simulink model "nms_model_nonlin"  (R2020a)
settings: Solver=VariableStepAuto  StartTime=0.0  StopTime=7  FixedStep=0.0001  MaxStep=.01  RelTol=1e-4  AbsTol=1e-6
values from neighbouring files (symbols this model uses):
  animFrameRate = 10    [runmodel.m]
  dt_visual = -1    [NMScontrol.m]    (also in runmodel.m = 0.001)
  g = params.g    [NMPCcostFunction.m]    (also in dynamicsNMPC.m = 9.81)
  m = parametersOpt(1)    [CGBgreybox.m]    (also in NMPCcostFunction.m = params.m)
  params = setupParamsStruct(parametersOpt, dt, controlParams)    [CGBcontrol.m]    (also in CGBgreybox.m = setupParamsStruct(parametersOpt); computationTime.m = setupParamsStruct(ParametersOpt, Qy, yref, dt))
undefined symbols (not defined in the file or in its folder): footMass, hatLeftHipToCenterDistWidth, hatMass, initialTargetAngle, legMass, LongDelay, LongLoopDelay, LPreStimBFSHinit, LPreStimGASinit, LPreStimGLUinit, LPreStimHABinit, LPreStimHADinit, LPreStimHAMinit, LPreStimHFLinit, LPreStimRFinit, LPreStimSOLinit, LPreStimTAinit, LPreStimVASinit, LTargetAngleInit, LTargetAngleRInit, MidDelay, RPreStimBFSHinit, RPreStimGASinit, RPreStimGLUinit, RPreStimHABinit, RPreStimHADinit, RPreStimHAMinit, RPreStimHFLinit, RPreStimRFinit, RPreStimSOLinit, RPreStimTAinit, RPreStimVASinit, RTargetAngleInit, RTargetAngleRInit, shankLength, shankMass, ShortDelay, termination_height, thetaHATref, thighLength, thighMass, totalMass, X, Y, Z
libraries: NeuroMuscularLibrary x113, nesl_utility x30, sm_lib x24, simulink x3
(part 3 of 5)

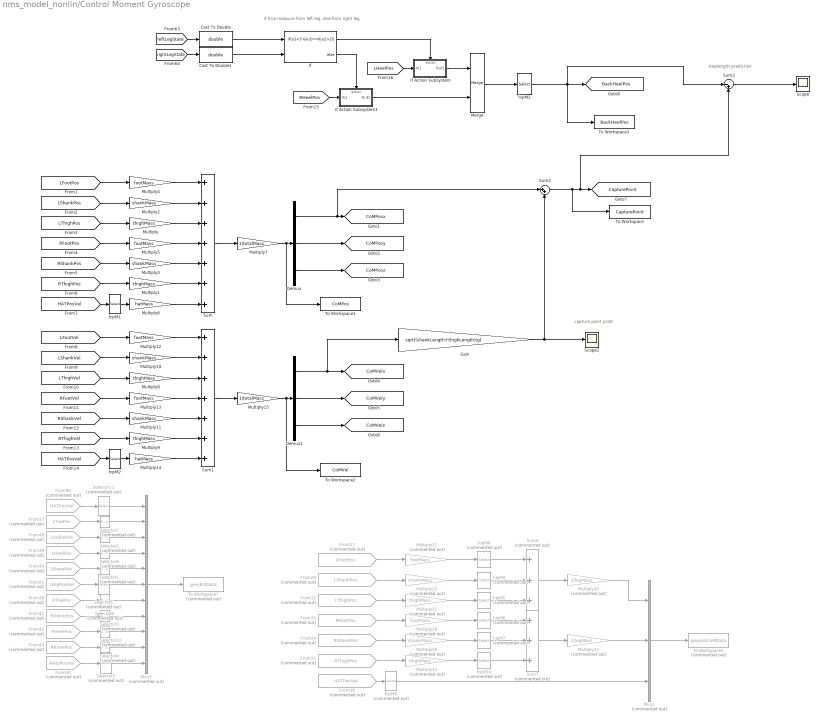
== system nms_model_nonlin/Control Moment Gyroscope ==
  note: capture point pratt
  note: steplength prediction
  note: if true measure from left leg, else from right leg
  Cast To Double : DataTypeConversion  OutDataTypeStr=double
  Cast To Double1 : DataTypeConversion  OutDataTypeStr=double
  Demux : Demux  Outputs=3
  Demux1 : Demux  Outputs=3
  From27 : From  Commented=on  GotoTag=LFootPos  TagVisibility=global
  From28 : From  Commented=on  GotoTag=LShankPos  TagVisibility=global
  From32 : From  Commented=on  GotoTag=LThighPos  TagVisibility=global
  From33 : From  Commented=on  GotoTag=RFootPos  TagVisibility=global
  From34 : From  Commented=on  GotoTag=RShankPos  TagVisibility=global
  From35 : From  Commented=on  GotoTag=RThighPos  TagVisibility=global
  From36 : From  Commented=on  GotoTag=HATPosVel  TagVisibility=global
  From37 : From  Commented=on  GotoTag=LToePos  TagVisibility=global
      settings: CloseFcn=tagdialog Close
  From38 : From  Commented=on  GotoTag=RToePos  TagVisibility=global
      settings: CloseFcn=tagdialog Close
  From39 : From  Commented=on  GotoTag=LHeelPos  TagVisibility=global
      settings: CloseFcn=tagdialog Close
  From40 : From  Commented=on  GotoTag=RHipPosVel  TagVisibility=global
  From41 : From  Commented=on  GotoTag=RAnklePos  TagVisibility=global
      settings: CloseFcn=tagdialog Close
  From42 : From  Commented=on  GotoTag=RHeelPos  TagVisibility=global
      settings: CloseFcn=tagdialog Close
  From43 : From  Commented=on  GotoTag=RKneePos  TagVisibility=global
      settings: CloseFcn=tagdialog Close
  From48 : From  Commented=on  GotoTag=LAnklePos  TagVisibility=global
      settings: CloseFcn=tagdialog Close
  From49 : From  Commented=on  GotoTag=LKneePos  TagVisibility=global
      settings: CloseFcn=tagdialog Close
  From90 : From  Commented=on  GotoTag=HATPosVel  TagVisibility=global
  From91 : From  Commented=on  GotoTag=LHipPosVel  TagVisibility=global
  Gain : Gain  Gain=sqrt((shankLength+thighLength)/g)
  If : If  NumInputs=2  IfExpression=u1<3 &(u2==0|u2>2)
  If Action Subsystem : Subsystem  TreatAsAtomicUnit=on
  If Action Subsystem1 : Subsystem  TreatAsAtomicUnit=on
  Merge : Merge
  Multiply{,1,8..9} (4 alike) : Gain  Gain=thighMass
  Multiply{2..3,10..11} (4 alike) : Gain  Gain=shankMass
  Multiply{4..5,12..13} (4 alike) : Gain  Gain=footMass
  Multiply14 : Gain  Gain=hatMass
  Multiply15 : Gain  Gain=1/totalMass
  Multiply25 : Gain  Commented=on  Gain=shankMass
  Multiply26 : Gain  Commented=on  Gain=shankMass
  Multiply27 : Gain  Commented=on  Gain=footMass
  Multiply28 : Gain  Commented=on  Gain=footMass
  Multiply30 : Gain  Commented=on  Gain=1/legMass
  Multiply31 : Gain  Commented=on  Gain=thighMass
  Multiply32 : Gain  Commented=on  Gain=thighMass
  Multiply33 : Gain  Commented=on  Gain=1/legMass
  Multiply6 : Gain  Gain=hatMass
  Multiply7 : Gain  Gain=1/totalMass
  Mux2 : Mux  Commented=on  Inputs=3
  Mux3 : Mux  Commented=on  Inputs=11
  Scope : Scope
  Scope1 : Scope
  Selector{1..4,7..10} (8 alike) : Selector  Commented=on  InputPortWidth=3  IndexOptions=Index vector (dialog)  Indices=[1 3]  OutputSizes=1
  Selector11 : Selector  Commented=on  InputPortWidth=6  IndexOptions=Index vector (dialog)  Indices=[1,3]  OutputSizes=1
  Selector5 : Selector  Commented=on  InputPortWidth=6  IndexOptions=Index vector (dialog)  Indices=[1,3]  OutputSizes=1
  Selector6 : Selector  Commented=on  InputPortWidth=6  IndexOptions=Index vector (dialog)  Indices=[1,3]  OutputSizes=1
  Sum : Sum  Inputs=+++++++
  Sum1 : Sum  Inputs=+++++++
  Sum2 : Sum  Inputs=|++
  Sum3 : Sum  Inputs=|-+
  Sum6 : Sum  Commented=on  Inputs=+++
  Sum7 : Sum  Commented=on  Inputs=+++
  To Workspace : ToWorkspace  VariableName=CapturePoint  SaveFormat=Structure With Time  SampleTime=0.01
  To Workspace1 : ToWorkspace  VariableName=CoMPos  SaveFormat=Structure With Time  SampleTime=0.01
  To Workspace2 : ToWorkspace  VariableName=CoMVel  SaveFormat=Structure With Time  SampleTime=0.01
  To Workspace3 : ToWorkspace  VariableName=BackHeelPos  SaveFormat=Structure With Time  SampleTime=0.01
  To Workspace5 : ToWorkspace  Commented=on  VariableName=greyEstCoMData  SaveFormat=Structure With Time  SampleTime=dt_visual
  To Workspace7 : ToWorkspace  Commented=on  VariableName=greyEstData  SaveFormat=Structure With Time  SampleTime=dt_visual
  hipM1 : Selector  InputPortWidth=6  IndexOptions=Index vector (dialog)  Indices=[1:3]  OutputSizes=1
  hipM{4..7,9..10} (6 alike) : Selector  Commented=on  InputPortWidth=3  IndexOptions=Index vector (dialog)  Indices=[1;3]  OutputSizes=1
  hipM2 : Selector  InputPortWidth=6  IndexOptions=Index vector (dialog)  Indices=[4:6]  OutputSizes=1
  hipM3 : Selector  InputPortWidth=3  IndexOptions=Index vector (dialog)  Indices=1  OutputSizes=1
  hipM8 : Selector  Commented=on  InputPortWidth=6  IndexOptions=Index vector (dialog)  Indices=[1;3]  OutputSizes=1
  tag scope: BackHeelPos=global, CapturePoint=global, CoMPosx=global, CoMPosy=global, CoMPosz=global, CoMVelx=global, CoMVely=global, CoMVelz=global
  wires:
  [LFootPos] -> Multiply4/1
  [LShankPos] -> Multiply2/1
  [RFootPos] -> Multiply5/1
  [LThighPos] -> Multiply/1
  [RShankPos] -> Multiply3/1
  [RThighPos] -> Multiply1/1
  [HATPosVel] -> hipM1/1
  Multiply4/1 -> Sum/1
  Multiply2/1 -> Sum/2
  Multiply/1 -> Sum/3
  Multiply5/1 -> Sum/4
  Multiply3/1 -> Sum/5
  Multiply1/1 -> Sum/6
  Multiply6/1 -> Sum/7
  Sum/1 -> Multiply7/1
  hipM1/1 -> Multiply6/1
  Multiply7/1 -> To Workspace1/1, Demux/1
  Demux/2 -> [CoMPosy]
  Demux/3 -> [CoMPosz]
  Demux/1 -> Sum2/1, [CoMPosx]
  Demux1/2 -> [CoMVely]
  hipM2/1 -> Multiply14/1
  Multiply14/1 -> Sum1/7
  Multiply12/1 -> Sum1/1
  Multiply8/1 -> Sum1/3
  [LThighVel] -> Multiply8/1
  [LShankVel] -> Multiply10/1
  Multiply13/1 -> Sum1/4
  [HATPosVel] -> hipM2/1
  Multiply11/1 -> Sum1/5
  Multiply15/1 -> To Workspace2/1, Demux1/1
  Multiply9/1 -> Sum1/6
  Demux1/3 -> [CoMVelz]
  [RFootVel] -> Multiply13/1
  Multiply10/1 -> Sum1/2
  [RThighVel] -> Multiply9/1
  Sum1/1 -> Multiply15/1
  [LFootVel] -> Multiply12/1
  [RShankVel] -> Multiply11/1
  Demux1/1 -> Gain/1, [CoMVelx]
  Gain/1 -> Sum2/2, Scope1/1
  Sum2/1 -> To Workspace/1, Sum3/2, [CapturePoint]
  [rightLegState] -> Cast To Double1/1
  [leftLegState] -> Cast To Double/1
  Cast To Double/1 -> If/1
  Cast To Double1/1 -> If/2
  If/1 -> If Action Subsystem/Action
  If/2 -> If Action Subsystem1/Action
  If Action Subsystem/1(Out1) -> Merge/1
  If Action Subsystem1/1(Out1) -> Merge/2
  [RHeelPos] -> If Action Subsystem1/1(In1)
  [LHeelPos] -> If Action Subsystem/1(In1)
  Merge/1 -> hipM3/1
  Sum3/1 -> Scope/1
  hipM3/1 -> Sum3/1, [BackHeelPos], To Workspace3/1
  hipM7/1 -> Sum7/2
  hipM8/1 -> Mux2/3
  hipM6/1 -> Sum7/1
  From33/1 -> Multiply28/1
  From35/1 -> Multiply32/1
  hipM9/1 -> Sum6/1
  From36/1 -> hipM8/1
  From32/1 -> Multiply31/1
  Multiply25/1 -> hipM4/1
  Multiply33/1 -> Mux2/2
  Sum6/1 -> Multiply30/1
  From28/1 -> Multiply25/1
  hipM4/1 -> Sum6/2
  Multiply27/1 -> hipM9/1
  From27/1 -> Multiply27/1
  Multiply31/1 -> hipM5/1
  Mux2/1 -> To Workspace5/1
  Sum7/1 -> Multiply33/1
  Multiply30/1 -> Mux2/1
  hipM5/1 -> Sum6/3
  hipM10/1 -> Sum7/3
  Multiply28/1 -> hipM6/1
  Multiply26/1 -> hipM7/1
  From34/1 -> Multiply26/1
  Multiply32/1 -> hipM10/1
  From40/1 -> Selector5/1
  From39/1 -> Selector9/1
  Selector9/1 -> Mux3/4
  Selector10/1 -> Mux3/9
  From42/1 -> Selector10/1
  From43/1 -> Selector4/1
  Selector5/1 -> Mux3/11
  Selector8/1 -> Mux3/7
  From48/1 -> Selector2/1
  Selector2/1 -> Mux3/3
  Selector6/1 -> Mux3/6
  Selector7/1 -> Mux3/2
  Selector11/1 -> Mux3/1
  Selector4/1 -> Mux3/10
  Selector3/1 -> Mux3/8
  From41/1 -> Selector3/1
  From37/1 -> Selector7/1
  From91/1 -> Selector6/1
  Mux3/1 -> To Workspace7/1
  From38/1 -> Selector8/1
  From90/1 -> Selector11/1
  From49/1 -> Selector1/1
  Selector1/1 -> Mux3/5

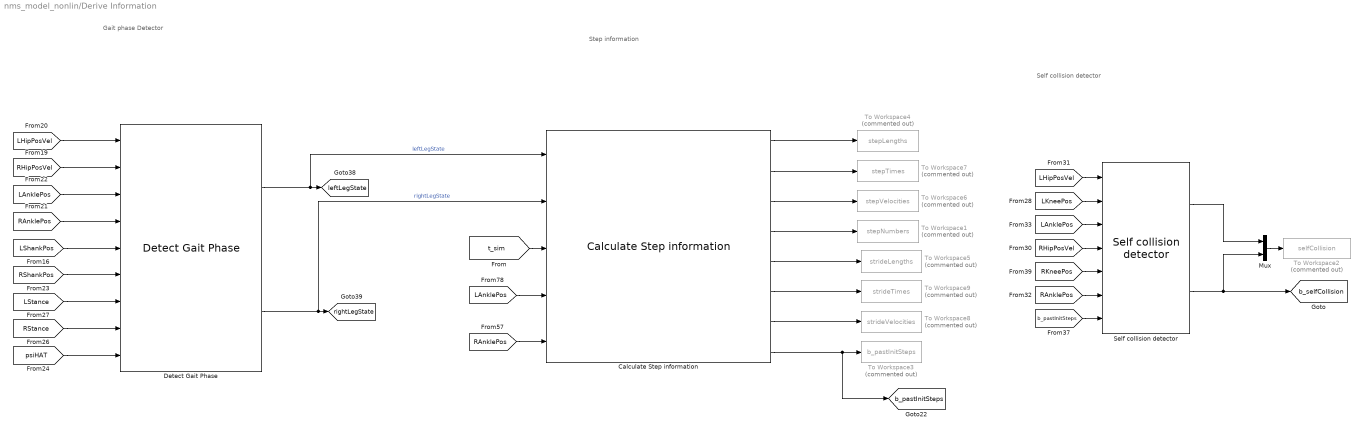
== system nms_model_nonlin/Derive Information ==
  note: Self collision detector
  note: Gait phase Detector
  note: Step information
  Calculate Step information : NeuroMuscularLibrary/Calculate Step information  initiationSteps=innerOptSettings.initiationSteps
  Detect Gait Phase : NeuroMuscularLibrary/Detect Gait Phase  SystemSampleTime=-1  Latency=0  AutoFrameSizeCalculation=off
  Mux : Mux  Inputs=2
  Self collision detector : NeuroMuscularLibrary/Self collision detector  maxDist=innerOptSettings.minLimbDistance
  To Workspace1 : ToWorkspace  Commented=on  VariableName=stepNumbers  SaveFormat=Structure With Time  SampleTime=-1
  To Workspace2 : ToWorkspace  Commented=on  VariableName=selfCollision  SaveFormat=Structure With Time  SampleTime=dt_visual
  To Workspace3 : ToWorkspace  Commented=on  VariableName=b_pastInitSteps  SaveFormat=Structure With Time  SampleTime=dt_visual
  To Workspace4 : ToWorkspace  Commented=on  VariableName=stepLengths  SaveFormat=Structure With Time  SampleTime=-1
  To Workspace5 : ToWorkspace  Commented=on  VariableName=strideLengths  SaveFormat=Structure With Time  SampleTime=-1
  To Workspace6 : ToWorkspace  Commented=on  VariableName=stepVelocities  SaveFormat=Structure With Time  SampleTime=-1
  To Workspace7 : ToWorkspace  Commented=on  VariableName=stepTimes  SaveFormat=Structure With Time  SampleTime=-1
  To Workspace8 : ToWorkspace  Commented=on  VariableName=strideVelocities  SaveFormat=Structure With Time  SampleTime=-1
  To Workspace9 : ToWorkspace  Commented=on  VariableName=strideTimes  SaveFormat=Structure With Time  SampleTime=-1
  tag scope: b_pastInitSteps=global, b_selfCollision=global, leftLegState=global, rightLegState=global
  wires:
  [RHipPosVel] -> Detect Gait Phase/2
  [LKneePos] -> Self collision detector/2
  [RHipPosVel] -> Self collision detector/4
  Mux/1 -> To Workspace2/1
  Self collision detector/2 -> [b_selfCollision], Mux/2
  [RAnklePos] -> Self collision detector/6
  Detect Gait Phase/1 -> Calculate Step information/1, [leftLegState]  "leftLegState"
  [LHipPosVel] -> Detect Gait Phase/1
  Self collision detector/1 -> Mux/1
  Detect Gait Phase/2 -> Calculate Step information/2, [rightLegState]  "rightLegState"
  [LHipPosVel] -> Self collision detector/1
  [b_pastInitSteps] -> Self collision detector/7
  [RStance] -> Detect Gait Phase/8
  [LStance] -> Detect Gait Phase/7
  [RShankPos] -> Detect Gait Phase/6
  [RAnklePos] -> Detect Gait Phase/4
  [psiHAT] -> Detect Gait Phase/9
  [RKneePos] -> Self collision detector/5
  [LAnklePos] -> Self collision detector/3
  [LShankPos] -> Detect Gait Phase/5
  [LAnklePos] -> Detect Gait Phase/3
  [RAnklePos] -> Calculate Step information/5
  Calculate Step information/1 -> To Workspace4/1
  Calculate Step information/3 -> To Workspace6/1
  [LAnklePos] -> Calculate Step information/4
  Calculate Step information/8 -> [b_pastInitSteps], To Workspace3/1
  Calculate Step information/4 -> To Workspace1/1
  [t_sim] -> Calculate Step information/3
  Calculate Step information/2 -> To Workspace7/1
  Calculate Step information/5 -> To Workspace5/1
  Calculate Step information/6 -> To Workspace9/1
  Calculate Step information/7 -> To Workspace8/1

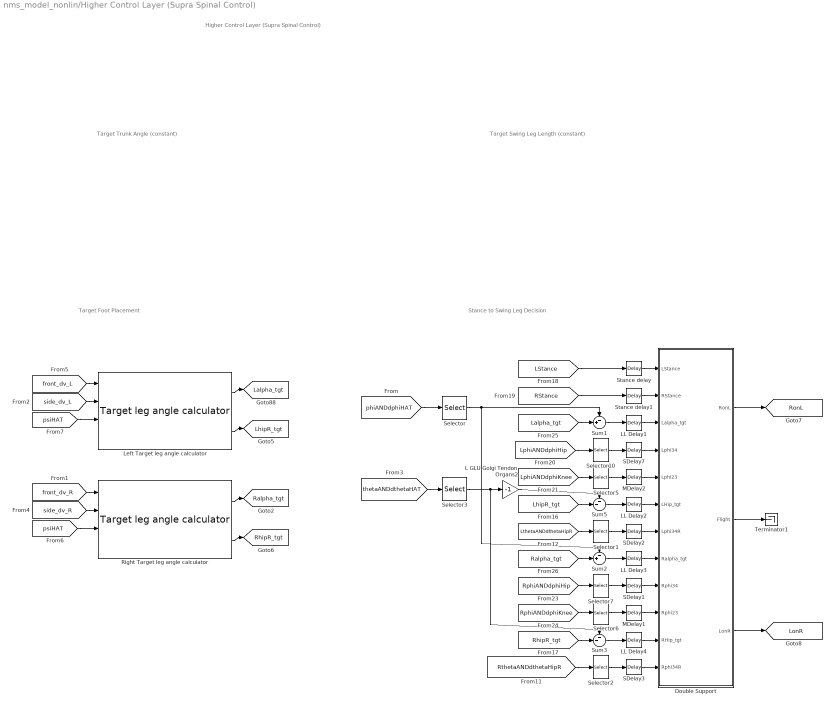
== system nms_model_nonlin/Higher Control Layer (Supra Spinal Control) ==
  note: Target Foot Placement
  note: Target Swing Leg Length
      | (constant)
  note: Stance to Swing Leg Decision
  note: Target Trunk Angle
      | (constant)
  note: Higher Control Layer
      | (Supra Spinal Control)
  Double Support : Subsystem
  L GLU Golgi Tendon Organs2 : Gain  Gain=-1
  LL Delay1 : TransportDelay  DelayTime=LongLoopDelay/2  InitialOutput=initialTargetAngle
  LL Delay2 : TransportDelay  DelayTime=LongLoopDelay/2
  LL Delay3 : TransportDelay  DelayTime=LongLoopDelay/2  InitialOutput=initialTargetAngle
  LL Delay4 : TransportDelay  DelayTime=LongLoopDelay/2
  Left Target leg angle calculator : NeuroMuscularLibrary/Target leg angle calculator  simbiconLegAngle0=simbiconLegAngle0  simbiconGainD=simbiconGainD  simbiconGainV=simbiconGainV  simbiconLegAngle0_C=simbiconLegAngle0_C  simbiconGainD_C=simbiconGainD_C  simbiconGainV_C=simbiconGainV_C  headingGain=0  headingIntGain=0
  MDelay1 : TransportDelay  DelayTime=MidDelay
  MDelay2 : TransportDelay  DelayTime=MidDelay
  Right Target leg angle calculator : NeuroMuscularLibrary/Target leg angle calculator  simbiconLegAngle0=simbiconLegAngle0  simbiconGainD=simbiconGainD  simbiconGainV=simbiconGainV  simbiconLegAngle0_C=simbiconLegAngle0_C  simbiconGainD_C=simbiconGainD_C  simbiconGainV_C=simbiconGainV_C  headingGain=0  headingIntGain=0
  SDelay{1..3,7} (4 alike) : TransportDelay  DelayTime=ShortDelay
  Selector : Selector  InputPortWidth=2  IndexOptions=Index vector (dialog)  Indices=[1]  OutputSizes=1
  Selector{1..2,5..7,10} (6 alike) : Selector  InputPortWidth=2  IndexOptions=Index vector (dialog)  Indices=1  OutputSizes=1
  Selector3 : Selector  InputPortWidth=2  IndexOptions=Index vector (dialog)  Indices=[1]  OutputSizes=1
  Stance delay : TransportDelay  DelayTime=MidDelay
  Stance delay1 : TransportDelay  DelayTime=MidDelay
  Sum1 : Sum  Inputs=-+|
  Sum2 : Sum  Inputs=-+|
  Sum3 : Sum  Inputs=--|
  Sum5 : Sum  Inputs=--|
  Terminator1 : Terminator
  tag scope: Lalpha_tgt=global, LhipR_tgt=global, LonR=global, Ralpha_tgt=global, RhipR_tgt=global, RonL=global
  wires:
  [LphiANDdphiHip] -> Selector10/1
  [LphiANDdphiKnee] -> Selector5/1
  Selector10/1 -> SDelay7/1
  Selector5/1 -> MDelay2/1
  [RphiANDdphiHip] -> Selector7/1
  [RphiANDdphiKnee] -> Selector6/1
  Selector7/1 -> SDelay1/1
  Selector6/1 -> MDelay1/1
  Double Support/3(LonR) -> [LonR]
  Stance delay/1 -> Double Support/1(LStance)
  Stance delay1/1 -> Double Support/2(RStance)
  Double Support/1(RonL) -> [RonL]
  [LStance] -> Stance delay/1
  [RStance] -> Stance delay1/1
  Double Support/2(Flight) -> Terminator1/1
  LL Delay1/1 -> Double Support/3(Lalpha_tgt)
  LL Delay3/1 -> Double Support/8(Ralpha_tgt)
  SDelay7/1 -> Double Support/4(Lphi34)
  SDelay1/1 -> Double Support/9(Rphi34)
  MDelay2/1 -> Double Support/5(Lphi23)
  MDelay1/1 -> Double Support/10(Rphi23)
  Sum1/1 -> LL Delay1/1
  [Lalpha_tgt] -> Sum1/2
  Selector/1 -> Sum2/1, Sum1/1
  [Ralpha_tgt] -> Sum2/2
  Sum2/1 -> LL Delay3/1
  [LthetaANDdthetaHipR] -> Selector1/1
  Selector1/1 -> SDelay2/1
  SDelay2/1 -> Double Support/7(Lphi34R)
  LL Delay2/1 -> Double Support/6(LHip_tgt)
  Sum5/1 -> LL Delay2/1
  [LhipR_tgt] -> Sum5/2
  Selector3/1 -> L GLU Golgi Tendon Organs2/1, Sum3/1
  L GLU Golgi Tendon Organs2/1 -> Sum5/1
  [RthetaANDdthetaHipR] -> Selector2/1
  Selector2/1 -> SDelay3/1
  SDelay3/1 -> Double Support/12(Rphi34R)
  LL Delay4/1 -> Double Support/11(RHip_tgt)
  Sum3/1 -> LL Delay4/1
  [RhipR_tgt] -> Sum3/2
  [phiANDdphiHAT] -> Selector/1
  [thetaANDdthetaHAT] -> Selector3/1
  Right Target leg angle calculator/2 -> [RhipR_tgt]
  Right Target leg angle calculator/1 -> [Ralpha_tgt]
  Left Target leg angle calculator/2 -> [LhipR_tgt]
  Left Target leg angle calculator/1 -> [Lalpha_tgt]
  [side_dv_R] -> Right Target leg angle calculator/2
  [side_dv_L] -> Left Target leg angle calculator/2
  [front_dv_R] -> Right Target leg angle calculator/1
  [front_dv_L] -> Left Target leg angle calculator/1
  [psiHAT] -> Right Target leg angle calculator/3
  [psiHAT] -> Left Target leg angle calculator/3

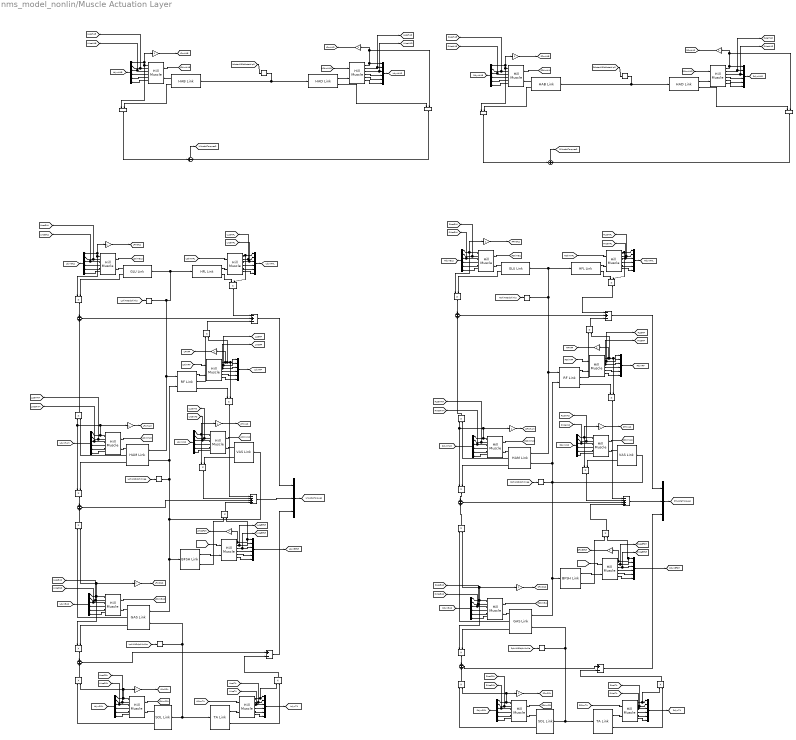
== system nms_model_nonlin/Muscle Actuation Layer ==
  note: Right Hip Joint
  note: Right Knee Joint
  note: Right Ankle Joint
  note: Left Hip Joint
  note: Left Knee Joint
  note: Left Ankle Joint
  note: Left Leg
  note: Right Leg
  note: Body Mechanics Layer
      | Interface (Left Hip Joint)
  note: Muscle Actuation Layer
      | (Coronal Plane)
  note: Muscle Actuation Layer
      | (Sagittal Plane)
  note: Body Mechanics Layer
      | Interface (Right Hip Joint)
  Add1 : Sum  Inputs=-+-
  Add2 : Sum  Inputs=-+-
  Add3 : Sum  Inputs=--++
  Add4 : Sum  Inputs=+-
  Add5 : Sum  Inputs=--++
  Add6 : Sum  Inputs=+-
  L  TA Link : NeuroMuscularLibrary/TA Link  SystemSampleTime=-1  Latency=0  AutoFrameSizeCalculation=off
  L BFSH Golgi Tendon Organs : Gain
  L BFSH Link : NeuroMuscularLibrary/BFSH Link  SystemSampleTime=-1  Latency=0  AutoFrameSizeCalculation=off
  L BFSH Muscle : NeuroMuscularLibrary/Hill Muscle  Fmax=FmaxBFSH  lopt=loptBFSH  vmax=vmaxBFSH  lslack=lslackBFSH
  L GAS Golgi Tendon Organs : Gain
  L GAS Link : NeuroMuscularLibrary/GAS Link  SystemSampleTime=-1  Latency=0  AutoFrameSizeCalculation=off
  L GAS Muscle : NeuroMuscularLibrary/Hill Muscle  Fmax=FmaxGAS  lopt=loptGAS  vmax=vmaxGAS  lslack=lslackGAS
  L GLU Golgi Tendon Organs : Gain
  L GLU Link : NeuroMuscularLibrary/GLU Link  SystemSampleTime=-1  Latency=0  AutoFrameSizeCalculation=off
  L GLU Muscle : NeuroMuscularLibrary/Hill Muscle  Fmax=FmaxGLU  lopt=loptGLU  vmax=vmaxGLU  lslack=lslackGLU
  L HAB Golgi Tendon Organs : Gain
  L HAB Link : NeuroMuscularLibrary/HAB Link  SystemSampleTime=-1  Latency=0  AutoFrameSizeCalculation=off
  L HAB Muscle : NeuroMuscularLibrary/Hill Muscle  Fmax=FmaxHAB  lopt=loptHAB  vmax=vmaxHAB  lslack=lslackHAB
  L HAD Golgi Tendon Organs : Gain
  L HAD Link : NeuroMuscularLibrary/HAD Link  SystemSampleTime=-1  Latency=0  AutoFrameSizeCalculation=off
  L HAD Muscle : NeuroMuscularLibrary/Hill Muscle  Fmax=FmaxHAD  lopt=loptHAD  vmax=vmaxHAD  lslack=lslackHAD
  L HAM Golgi Tendon Organs : Gain
  L HAM Link : NeuroMuscularLibrary/HAM Link  SystemSampleTime=-1  Latency=0  AutoFrameSizeCalculation=off
  L HAM Muscle : NeuroMuscularLibrary/Hill Muscle  Fmax=FmaxHAM  lopt=loptHAM  vmax=vmaxHAM  lslack=lslackHAM
  L HFL Link : NeuroMuscularLibrary/HFL Link  SystemSampleTime=-1  Latency=0  AutoFrameSizeCalculation=off
  L HFL Muscle : NeuroMuscularLibrary/Hill Muscle  Fmax=FmaxHFL  lopt=loptHFL  vmax=vmaxHFL  lslack=lslackHFL
  L RF Golgi Tendon Organs : Gain
  L RF Link : NeuroMuscularLibrary/RF Link  SystemSampleTime=-1  Latency=0  AutoFrameSizeCalculation=off
  L RF Muscle : NeuroMuscularLibrary/Hill Muscle  Fmax=FmaxRF  lopt=loptRF  vmax=vmaxRF  lslack=lslackRF
  L SOL Golgi Tendon Organs : Gain
  L SOL Link : NeuroMuscularLibrary/SOL Link  SystemSampleTime=-1  Latency=0  AutoFrameSizeCalculation=off
  L SOL Muscle : NeuroMuscularLibrary/Hill Muscle  Fmax=FmaxSOL  lopt=loptSOL  vmax=vmaxSOL  lslack=lslackSOL
  L TA Muscle : NeuroMuscularLibrary/Hill Muscle  Fmax=FmaxTA  lopt=loptTA  vmax=vmaxTA  lslack=lslackTA
  L VAS Golgi Tendon Organs : Gain
  L VAS Link : NeuroMuscularLibrary/VAS Link  SystemSampleTime=-1  Latency=0  AutoFrameSizeCalculation=off
  L VAS Muscle : NeuroMuscularLibrary/Hill Muscle  Fmax=FmaxVAS  lopt=loptVAS  vmax=vmaxVAS  lslack=lslackVAS
  Mux : Mux  Inputs=3
  Mux1 : Mux  Inputs=3
  Mux{2..23} (22 alike) : Mux  Inputs=6
  Product{1..2,26..27} (4 alike) : Product  RndMeth=Zero
  R  TA Link : NeuroMuscularLibrary/TA Link  SystemSampleTime=-1  Latency=0  AutoFrameSizeCalculation=off
  R BFSH Golgi Tendon Organs : Gain
  R BFSH Link : NeuroMuscularLibrary/BFSH Link  SystemSampleTime=-1  Latency=0  AutoFrameSizeCalculation=off
  R BFSH Muscle : NeuroMuscularLibrary/Hill Muscle  Fmax=FmaxBFSH  lopt=loptBFSH  vmax=vmaxBFSH  lslack=lslackBFSH
  R GAS Golgi Tendon Organs : Gain
  R GAS Link : NeuroMuscularLibrary/GAS Link  SystemSampleTime=-1  Latency=0  AutoFrameSizeCalculation=off
  R GAS Muscle : NeuroMuscularLibrary/Hill Muscle  Fmax=FmaxGAS  lopt=loptGAS  vmax=vmaxGAS  lslack=lslackGAS
  R GLU Golgi Tendon Organs : Gain
  R GLU Link : NeuroMuscularLibrary/GLU Link  SystemSampleTime=-1  Latency=0  AutoFrameSizeCalculation=off
  R GLU Muscle : NeuroMuscularLibrary/Hill Muscle  Fmax=FmaxGLU  lopt=loptGLU  vmax=vmaxGLU  lslack=lslackGLU
  R HAB Golgi Tendon Organs : Gain
  R HAB Link : NeuroMuscularLibrary/HAB Link  SystemSampleTime=-1  Latency=0  AutoFrameSizeCalculation=off
  R HAB Muscle : NeuroMuscularLibrary/Hill Muscle  Fmax=FmaxHAB  lopt=loptHAB  vmax=vmaxHAB  lslack=lslackHAB
  R HAD Golgi Tendon Organs : Gain
  R HAD Link : NeuroMuscularLibrary/HAD Link  SystemSampleTime=-1  Latency=0  AutoFrameSizeCalculation=off
  R HAD Muscle : NeuroMuscularLibrary/Hill Muscle  Fmax=FmaxHAD  lopt=loptHAD  vmax=vmaxHAD  lslack=lslackHAD
  R HAM Golgi Tendon Organs : Gain
  R HAM Link : NeuroMuscularLibrary/HAM Link  SystemSampleTime=-1  Latency=0  AutoFrameSizeCalculation=off
  R HAM Muscle : NeuroMuscularLibrary/Hill Muscle  Fmax=FmaxHAM  lopt=loptHAM  vmax=vmaxHAM  lslack=lslackHAM
  R HFL Link : NeuroMuscularLibrary/HFL Link  SystemSampleTime=-1  Latency=0  AutoFrameSizeCalculation=off
  R HFL Muscle : NeuroMuscularLibrary/Hill Muscle  Fmax=FmaxHFL  lopt=loptHFL  vmax=vmaxHFL  lslack=lslackHFL
  R RF Golgi Tendon Organs : Gain
  R RF Link : NeuroMuscularLibrary/RF Link  SystemSampleTime=-1  Latency=0  AutoFrameSizeCalculation=off
  R RF Muscle : NeuroMuscularLibrary/Hill Muscle  Fmax=FmaxRF  lopt=loptRF  vmax=vmaxRF  lslack=lslackRF
  R SOL Golgi Tendon Organs : Gain
  R SOL Link : NeuroMuscularLibrary/SOL Link  SystemSampleTime=-1  Latency=0  AutoFrameSizeCalculation=off
  R SOL Muscle : NeuroMuscularLibrary/Hill Muscle  Fmax=FmaxSOL  lopt=loptSOL  vmax=vmaxSOL  lslack=lslackSOL
  R TA Muscle : NeuroMuscularLibrary/Hill Muscle  Fmax=FmaxTA  lopt=loptTA  vmax=vmaxTA  lslack=lslackTA
  R VAS Golgi Tendon Organs : Gain
  R VAS Link : NeuroMuscularLibrary/VAS Link  SystemSampleTime=-1  Latency=0  AutoFrameSizeCalculation=off
  R VAS Muscle : NeuroMuscularLibrary/Hill Muscle  Fmax=FmaxVAS  lopt=loptVAS  vmax=vmaxVAS  lslack=lslackVAS
  Selector{1..8} (8 alike) : Selector  InputPortWidth=2  IndexOptions=Index vector (dialog)  Indices=1  OutputSizes=1
  Sum{1,3..4,8,11,15} (6 alike) : Sum  Inputs=+|+
  Sum2 : Sum  Inputs=+-
  Sum25 : Sum  Inputs=+-
  tau = r*F{1..24} (24 alike) : Product
  tag scope: LFmBFSH=global, LFmGAS=global, LFmGLU=global, LFmHAB=global, LFmHAD=global, LFmHAM=global, LFmRF=global, LFmSOL=global, LFmVAS=global, LLceBFSH=global, LLceGAS=global, LLceGLU=global, LLceHAB=global, LLceHAD=global, LLceHAM=global, LLceHFL=global, LLceRF=global, LLceSOL=global, LLceTA=global, LLceVAS=global, LMuscleTorques=global, LMuscleTorquesR=global, LVceBFSH=global, LVceGAS=global, LVceGLU=global, LVceHAB=global, LVceHAD=global, LVceHAM=global, LVceHFL=global, LVceRF=global, LVceSOL=global, LVceTA=global, LVceVAS=global, LdynBFSH=global, LdynGAS=global, LdynGLU=global, LdynHAB=global, LdynHAD=global, LdynHAM=global, LdynHFL=global, LdynRF=global, LdynSOL=global, LdynTA=global, LdynVAS=global, RFmBFSH=global, RFmGAS=global, RFmGLU=global, RFmHAB=global, RFmHAD=global, RFmHAM=global, RFmRF=global, RFmSOL=global, RFmVAS=global, RLceBFSH=global, RLceGAS=global, RLceGLU=global, RLceHAB=global, RLceHAD=global, RLceHAM=global, RLceHFL=global, RLceRF=global, RLceSOL=global, RLceTA=global, RLceVAS=global, RMuscleTorques=global, RMuscleTorquesR=global, RVceBFSH=global, RVceGAS=global, RVceGLU=global, RVceHAB=global, RVceHAD=global, RVceHAM=global, RVceHFL=global, RVceRF=global, RVceSOL=global, RVceTA=global, RVceVAS=global, RdynBFSH=global, RdynGAS=global, RdynGLU=global, RdynHAB=global, RdynHAD=global, RdynHAM=global, RdynHFL=global, RdynRF=global, RdynSOL=global, RdynTA=global, RdynVAS=global
  wires:
  R HAM Link/1 -> R HAM Muscle/2
  R HAM Link/2 -> tau = r*F9/2
  R HAM Muscle/5 -> Mux7/5
  Mux7/1 -> [RdynHAM]
  R HAM Muscle/3 -> [RVceHAM], Mux7/3
  R HAM Muscle/4 -> Mux7/4
  [RphiANDdphiHip] -> Selector1/1
  Selector1/1 -> R RF Link/1, R HAM Link/1, R GLU Link/1, R HFL Link/1
  Add2/1 -> Mux/1
  R GLU Link/1 -> R GLU Muscle/2
  [RStimGLU] -> R GLU Muscle/1
  R GLU Muscle/5 -> Mux9/5
  R GLU Muscle/2 -> [RLceGLU], Mux9/2
  R GLU Muscle/3 -> [RVceGLU], Mux9/3
  R GLU Muscle/4 -> Mux9/4
  R GLU Link/2 -> tau = r*F10/2
  R GLU Muscle/1 -> Mux9/1, R GLU Golgi Tendon Organs/1, tau = r*F10/1
  R GLU Golgi Tendon Organs/1 -> [RFmGLU]
  R HFL Link/1 -> R HFL Muscle/2
  [RStimHFL] -> R HFL Muscle/1
  R HFL Muscle/5 -> Mux10/5
  Mux10/1 -> [RdynHFL]
  R HFL Muscle/4 -> Mux10/4
  R HFL Muscle/3 -> [RVceHFL], Mux10/3
  R HFL Link/2 -> tau = r*F11/1
  R HFL Muscle/1 -> Mux10/1, tau = r*F11/2
  R HAM Golgi Tendon Organs/1 -> [RFmHAM]
  [RStimHAM] -> R HAM Muscle/1
  R VAS Link/1 -> R VAS Muscle/2
  R VAS Muscle/5 -> Mux11/5
  Mux11/1 -> [RdynVAS]
  R VAS Muscle/2 -> [RLceVAS], Mux11/2
  R VAS Muscle/3 -> [RVceVAS], Mux11/3
  R VAS Muscle/4 -> Mux11/4
  R VAS Muscle/1 -> R VAS Golgi Tendon Organs/1, Mux11/1, tau = r*F13/1
  R VAS Golgi Tendon Organs/1 -> [RFmVAS]
  R VAS Link/2 -> tau = r*F13/2
  R HAM Link/3 -> tau = r*F14/2
  Sum11/1 -> Add3/3  "Knee Flexion Torque"
  [RStimVAS] -> R VAS Muscle/1
  [RphiANDdphiKnee] -> Selector3/1
  R SOL Muscle/1 -> R SOL Golgi Tendon Organs/1, tau = r*F12/2, Mux13/1
  R SOL Muscle/5 -> Mux13/5
  Mux13/1 -> [RdynSOL]
  R SOL Muscle/2 -> [RLceSOL], Mux13/2
  R SOL Muscle/3 -> [RVceSOL], Mux13/3
  R SOL Muscle/4 -> Mux13/4
  R SOL Link/2 -> tau = r*F12/1
  R SOL Link/1 -> R SOL Muscle/2
  R SOL Golgi Tendon Organs/1 -> [RFmSOL]
  [RStimSOL] -> R SOL Muscle/1
  Selector2/1 -> R GAS Link/2, R  TA Link/1, R SOL Link/1
  [RphiANDdphiAnkle] -> Selector2/1
  Add4/1 -> Mux/3
  R  TA Link/1 -> R TA Muscle/2
  R TA Muscle/1 -> tau = r*F15/1, Mux14/1
  R TA Muscle/5 -> Mux14/5
  Mux14/1 -> [RdynTA]
  R TA Muscle/4 -> Mux14/4
  R TA Muscle/3 -> Mux14/3, [RVceTA]
  [RStimTA] -> R TA Muscle/1
  R  TA Link/2 -> tau = r*F15/2
  tau = r*F15/1 -> Add4/2
  R GAS Link/1 -> R GAS Muscle/2
  Selector3/1 -> R RF Link/2, R HAM Link/2, R VAS Link/1, R GAS Link/1, R BFSH Link/1
  R GAS Muscle/5 -> Mux12/5
  Mux12/1 -> [RdynGAS]
  R GAS Muscle/2 -> [RLceGAS], Mux12/2
  R GAS Muscle/3 -> [RVceGAS], Mux12/3
  R GAS Muscle/4 -> Mux12/4
  R GAS Link/2 -> tau = r*F16/1
  [RStimGAS] -> R GAS Muscle/1
  tau = r*F12/1 -> Sum15/2
  Sum15/1 -> Add4/1
  R GAS Link/3 -> tau = r*F17/2
  tau = r*F17/1 -> Sum15/1
  R GAS Muscle/1 -> Mux12/1, tau = r*F16/2, R GAS Golgi Tendon Organs/1, tau = r*F17/1
  R GAS Golgi Tendon Organs/1 -> [RFmGAS]
  tau = r*F9/1 -> Sum8/2  "HAM"
  tau = r*F10/1 -> Sum8/1  "GLU"
  tau = r*F11/1 -> Add2/1  "HFL"
  R HAM Muscle/1 -> tau = r*F14/1, tau = r*F9/1, R HAM Golgi Tendon Organs/1, Mux7/1
  Sum8/1 -> Add2/2  "Hip Extension Moment"
  tau = r*F16/1 -> Sum11/2  "GAS"
  tau = r*F14/1 -> Sum11/1  "HAM"
  tau = r*F13/1 -> Add3/2  "VAS"
  R TA Muscle/2 -> [RLceTA], Mux14/2
  Mux9/1 -> [RdynGLU]
  Mux/1 -> [RMuscleTorques]
  L HAM Link/1 -> L HAM Muscle/2
  L HAM Link/2 -> tau = r*F18/2
  L HAM Muscle/5 -> Mux8/5
  Mux8/1 -> [LdynHAM]
  L HAM Muscle/3 -> [LVceHAM], Mux8/3
  L HAM Muscle/4 -> Mux8/4
  [LphiANDdphiHip] -> Selector4/1
  Selector4/1 -> L GLU Link/1, L HFL Link/1, L RF Link/1, L HAM Link/1
  Add1/1 -> Mux1/1
  L GLU Link/1 -> L GLU Muscle/2
  [LStimGLU] -> L GLU Muscle/1
  L GLU Muscle/5 -> Mux15/5
  L GLU Muscle/2 -> Mux15/2, [LLceGLU]
  L GLU Muscle/3 -> Mux15/3, [LVceGLU]
  L GLU Muscle/4 -> Mux15/4
  L GLU Link/2 -> tau = r*F1/2
  L GLU Muscle/1 -> Mux15/1, L GLU Golgi Tendon Organs/1, tau = r*F1/1
  L GLU Golgi Tendon Organs/1 -> [LFmGLU]
  L HFL Link/1 -> L HFL Muscle/2
  [LStimHFL] -> L HFL Muscle/1
  L HFL Muscle/5 -> Mux2/5
  Mux2/1 -> [LdynHFL]
  L HFL Muscle/4 -> Mux2/4
  L HFL Muscle/3 -> [LVceHFL], Mux2/3
  L HFL Link/2 -> tau = r*F2/1
  L HFL Muscle/1 -> Mux2/1, tau = r*F2/2
  L HAM Golgi Tendon Organs/1 -> [LFmHAM]
  [LStimHAM] -> L HAM Muscle/1
  L VAS Link/1 -> L VAS Muscle/2
  L VAS Muscle/5 -> Mux3/5
  Mux3/1 -> [LdynVAS]
  L VAS Muscle/2 -> [LLceVAS], Mux3/2
  L VAS Muscle/3 -> [LVceVAS], Mux3/3
  L VAS Muscle/4 -> Mux3/4
  L VAS Muscle/1 -> L VAS Golgi Tendon Organs/1, Mux3/1, tau = r*F4/1
  L VAS Golgi Tendon Organs/1 -> [LFmVAS]
  L VAS Link/2 -> tau = r*F4/2
  L HAM Link/3 -> tau = r*F5/2
  Sum1/1 -> Add5/3  "Knee Flexion Torque"
  [LStimVAS] -> L VAS Muscle/1
  [LphiANDdphiKnee] -> Selector6/1
  L SOL Muscle/1 -> L SOL Golgi Tendon Organs/1, tau = r*F3/2, Mux5/1
  L SOL Muscle/5 -> Mux5/5
  Mux5/1 -> [LdynSOL]
  L SOL Muscle/3 -> [LVceSOL], Mux5/3
  L SOL Muscle/4 -> Mux5/4
  L SOL Link/2 -> tau = r*F3/1
  L SOL Link/1 -> L SOL Muscle/2
  L SOL Golgi Tendon Organs/1 -> [LFmSOL]
  [LStimSOL] -> L SOL Muscle/1
  Selector5/1 -> L GAS Link/2, L  TA Link/1, L SOL Link/1
  [LphiANDdphiAnkle] -> Selector5/1
  Add6/1 -> Mux1/3
  L  TA Link/1 -> L TA Muscle/2
  L TA Muscle/1 -> tau = r*F6/1, Mux6/1
  L TA Muscle/5 -> Mux6/5
  Mux6/1 -> [LdynTA]
  L TA Muscle/4 -> Mux6/4
  L TA Muscle/3 -> Mux6/3, [LVceTA]
  [LStimTA] -> L TA Muscle/1
  L  TA Link/2 -> tau = r*F6/2
  tau = r*F6/1 -> Add6/2
  L GAS Link/1 -> L GAS Muscle/2
  Selector6/1 -> L GAS Link/1, L BFSH Link/1, L VAS Link/1, L RF Link/2, L HAM Link/2
  L GAS Muscle/5 -> Mux4/5
  Mux4/1 -> [LdynGAS]
  L GAS Muscle/2 -> [LLceGAS], Mux4/2
  L GAS Muscle/3 -> [LVceGAS], Mux4/3
  L GAS Muscle/4 -> Mux4/4
  L GAS Link/2 -> tau = r*F7/1
  [LStimGAS] -> L GAS Muscle/1
  tau = r*F3/1 -> Sum3/2
  Sum3/1 -> Add6/1
  L GAS Link/3 -> tau = r*F8/2
  tau = r*F8/1 -> Sum3/1
  L GAS Muscle/1 -> Mux4/1, tau = r*F7/2, L GAS Golgi Tendon Organs/1, tau = r*F8/1
  L GAS Golgi Tendon Organs/1 -> [LFmGAS]
  tau = r*F18/1 -> Sum4/2  "HAM"
  tau = r*F1/1 -> Sum4/1  "GLU"
  tau = r*F2/1 -> Add1/1  "HFL"
  L HAM Muscle/1 -> tau = r*F5/1, tau = r*F18/1, L HAM Golgi Tendon Organs/1, Mux8/1
  Sum4/1 -> Add1/2  "Hip Extension Moment"
  tau = r*F7/1 -> Sum1/2  "GAS"
  tau = r*F5/1 -> Sum1/1  "HAM"
  tau = r*F4/1 -> Add5/2  "VAS"
  L TA Muscle/2 -> [LLceTA], Mux6/2
  Mux15/1 -> [LdynGLU]
  Mux1/1 -> [LMuscleTorques]
  L GLU Muscle/6 -> Mux15/6
  L HFL Muscle/6 -> Mux2/6
  L HAM Muscle/6 -> Mux8/6
  L VAS Muscle/6 -> Mux3/6
  L GAS Muscle/6 -> Mux4/6
  L SOL Muscle/6 -> Mux5/6
  L TA Muscle/6 -> Mux6/6
  R SOL Muscle/6 -> Mux13/6
  R TA Muscle/6 -> Mux14/6
  R GAS Muscle/6 -> Mux12/6
  R HAM Muscle/6 -> Mux7/6
  R VAS Muscle/6 -> Mux11/6
  R HFL Muscle/6 -> Mux10/6
  R GLU Muscle/6 -> Mux9/6
  R HFL Muscle/2 -> [RLceHFL], Mux10/2
  R HAM Muscle/2 -> [RLceHAM], Mux7/2
  L HFL Muscle/2 -> [LLceHFL], Mux2/2
  L HAM Muscle/2 -> [LLceHAM], Mux8/2
  L SOL Muscle/2 -> [LLceSOL], Mux5/2
  L BFSH Muscle/3 -> [LVceBFSH], Mux16/3
  [LStimBFSH] -> L BFSH Muscle/1
  L BFSH Link/2 -> tau = r*F19/1
  L BFSH Golgi Tendon Organs/1 -> [LFmBFSH]
  L BFSH Muscle/6 -> Mux16/6
  L BFSH Muscle/4 -> Mux16/4
  L BFSH Link/1 -> L BFSH Muscle/2
  Mux16/1 -> [LdynBFSH]
  L BFSH Muscle/2 -> [LLceBFSH], Mux16/2
  L BFSH Muscle/5 -> Mux16/5
  L BFSH Muscle/1 -> tau = r*F19/2, Mux16/1, L BFSH Golgi Tendon Organs/1
  tau = r*F19/1 -> Add5/4  "BFSH"
  L RF Muscle/3 -> [LVceRF], Mux17/3
  [LStimRF] -> L RF Muscle/1
  L RF Link/3 -> tau = r*F20/2
  L RF Golgi Tendon Organs/1 -> [LFmRF]
  L RF Muscle/6 -> Mux17/6
  L RF Muscle/4 -> Mux17/4
  L RF Link/1 -> L RF Muscle/2
  Mux17/1 -> [LdynRF]
  L RF Muscle/2 -> [LLceRF], Mux17/2
  L RF Muscle/5 -> Mux17/5
  L RF Muscle/1 -> tau = r*F21/2, Mux17/1, tau = r*F20/1, L RF Golgi Tendon Organs/1
  L RF Link/2 -> tau = r*F21/1
  tau = r*F21/1 -> Add1/3  "RF"
  tau = r*F20/1 -> Add5/1  "RF"
  R BFSH Muscle/3 -> [RVceBFSH], Mux18/3
  [RStimBFSH] -> R BFSH Muscle/1
  R BFSH Muscle/1 -> tau = r*F22/2, Mux18/1, R BFSH Golgi Tendon Organs/1
  R BFSH Muscle/4 -> Mux18/4
  R BFSH Golgi Tendon Organs/1 -> [RFmBFSH]
  R BFSH Muscle/5 -> Mux18/5
  Mux18/1 -> [RdynBFSH]
  R BFSH Muscle/2 -> [RLceBFSH], Mux18/2
  R BFSH Link/1 -> R BFSH Muscle/2
  R BFSH Link/2 -> tau = r*F22/1
  R BFSH Muscle/6 -> Mux18/6
  tau = r*F22/1 -> Add3/4  "BFSH"
  [RStimRF] -> R RF Muscle/1
  R RF Muscle/3 -> [RVceRF], Mux19/3
  R RF Muscle/4 -> Mux19/4
  R RF Muscle/6 -> Mux19/6
  R RF Muscle/5 -> Mux19/5
  R RF Muscle/2 -> [RLceRF], Mux19/2
  R RF Muscle/1 -> tau = r*F24/2, Mux19/1, tau = r*F23/1, R RF Golgi Tendon Organs/1
  Mux19/1 -> [RdynRF]
  R RF Link/3 -> tau = r*F23/2
  R RF Link/2 -> tau = r*F24/1
  R RF Golgi Tendon Organs/1 -> [RFmRF]
  R RF Link/1 -> R RF Muscle/2
  tau = r*F24/1 -> Add2/3  "RF"
  tau = r*F23/1 -> Add3/1  "RF"
  Product27/1 -> Sum25/2
  L HAD Link/2 -> Product27/1
  Selector7/1 -> L HAB Link/1, L HAD Link/1
  Product26/1 -> Sum25/1
  L HAB Muscle/6 -> Mux20/6
  L HAB Muscle/1 -> Product26/1, Mux20/1, L HAB Golgi Tendon Organs/1
  L HAB Golgi Tendon Organs/1 -> [LFmHAB]
  L HAB Muscle/4 -> Mux20/4
  L HAB Muscle/2 -> Mux20/2, [LLceHAB]
  L HAB Muscle/5 -> Mux20/5
  L HAB Link/1 -> L HAB Muscle/2
  L HAB Link/2 -> Product26/2
  L HAB Muscle/3 -> Mux20/3, [LVceHAB]
  [LStimHAB] -> L HAB Muscle/1
  Mux20/1 -> [LdynHAB]
  [LthetaANDdthetaHipR] -> Selector7/1
  L HAD Link/1 -> L HAD Muscle/2
  [LStimHAD] -> L HAD Muscle/1
  L HAD Golgi Tendon Organs/1 -> [LFmHAD]
  L HAD Muscle/2 -> Mux21/2, [LLceHAD]
  L HAD Muscle/1 -> Mux21/1, Product27/2, L HAD Golgi Tendon Organs/1
  L HAD Muscle/3 -> [LVceHAD], Mux21/3
  L HAD Muscle/4 -> Mux21/4
  L HAD Muscle/5 -> Mux21/5
  L HAD Muscle/6 -> Mux21/6
  Mux21/1 -> [LdynHAD]
  Sum25/1 -> [LMuscleTorquesR]
  R HAD Muscle/6 -> Mux23/6
  Selector8/1 -> R HAB Link/1, R HAD Link/1
  R HAD Link/2 -> Product2/1
  R HAD Golgi Tendon Organs/1 -> [RFmHAD]
  [RStimHAD] -> R HAD Muscle/1
  Mux23/1 -> [RdynHAD]
  Sum2/1 -> [RMuscleTorquesR]
  Mux22/1 -> [RdynHAB]
  R HAB Golgi Tendon Organs/1 -> [RFmHAB]
  Product1/1 -> Sum2/1
  Product2/1 -> Sum2/2
  R HAD Muscle/5 -> Mux23/5
  R HAD Muscle/2 -> Mux23/2, [RLceHAD]
  R HAD Muscle/3 -> [RVceHAD], Mux23/3
  R HAD Link/1 -> R HAD Muscle/2
  [RthetaANDdthetaHipR] -> Selector8/1
  R HAD Muscle/1 -> Mux23/1, Product2/2, R HAD Golgi Tendon Organs/1
  R HAB Link/2 -> Product1/2
  R HAB Muscle/5 -> Mux22/5
  R HAB Muscle/2 -> Mux22/2, [RLceHAB]
  R HAD Muscle/4 -> Mux23/4
  R HAB Link/1 -> R HAB Muscle/2
  R HAB Muscle/4 -> Mux22/4
  R HAB Muscle/3 -> Mux22/3, [RVceHAB]
  R HAB Muscle/6 -> Mux22/6
  R HAB Muscle/1 -> Product1/1, Mux22/1, R HAB Golgi Tendon Organs/1
  [RStimHAB] -> R HAB Muscle/1
  Add5/1 -> Mux1/2
  Add3/1 -> Mux/2
